simulink model "Vehicle_Speedometer_Module"  (R2022a)
settings: Solver=FixedStepDiscrete  StartTime=0.0  StopTime=10.0  FixedStep=0.01  RelTol=1e-3
libraries: simulink x1
settings Model: DataDictionary=VSM_Data_Dictionary.sldd  EnableAccessToBaseWorkspace=off  Creator=jamesbond  LastModifiedBy=jamesbond
settings OptimizationCC: DefaultParameterBehavior=Inlined  EnhancedBackFolding=on  PassReuseOutputArgsAs=Individual arguments  ZeroExternalMemoryAtStartup=off  ZeroInternalMemoryAtStartup=off  OptimizeBlockOrder=speed  DifferentSizesBufferReuse=on  OptimizationCustomize=off  EfficientTunableParamExpr=on
settings DebuggingCC: SignalInfNanChecking=error  SignalRangeChecking=warning  CheckMatrixSingularityMsg=error  IntegerOverflowMsg=none  ParameterOverflowMsg=none  ParameterTunabilityLossMsg=error  ModelReferenceVersionMismatchMessage=warning  ModelReferenceIOMismatchMessage=warning  IntegerSaturationMsg=none
settings HardwareCC: ProdBitPerLong=64  ProdHWDeviceType=Intel->x86-64 (Mac OS X)
settings SFSimCC: MATLABDynamicMemAlloc=off
settings RTWCC: SystemTargetFile=ert.tlc  TemplateMakefile=ert_default_tmf  GenerateReport=on  LaunchReport=on  GenerateCodeMetricsReport=on
settings CodeAppCC: ForceParamTrailComments=on  IgnoreCustomStorageClasses=off  OperatorAnnotations=on  SimulinkDataObjDesc=on  SFDataObjDesc=on  InsertBlockDesc=on
settings ERTTargetCC: TargetLangStandard=C99 (ISO)  GenerateSampleERTMain=on  InlinedParameterPlacement=NonHierarchical  ERTCustomFileTemplate=example_file_process.tlc
settings ConfigComp: DVMaxProcessTime=3000  DVModelCoverageObjectives=MCDC  DVTestSuiteOptimization=Auto  DVDetectDeadLogic=on  DVDetectOutOfBounds=on  DVModelReferenceHarness=on  DVHarnessSource=Signal Editor

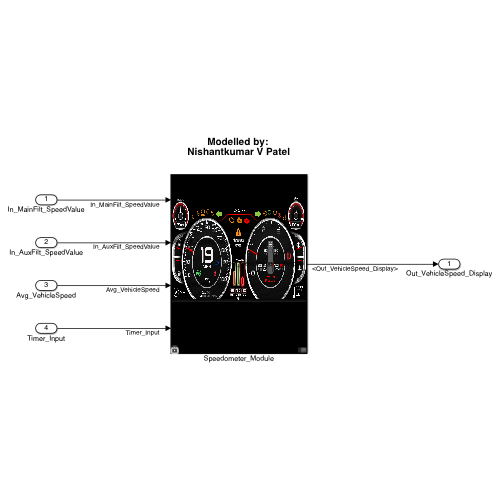
[thumbnail: Simulink's stored preview of the top-level diagram]
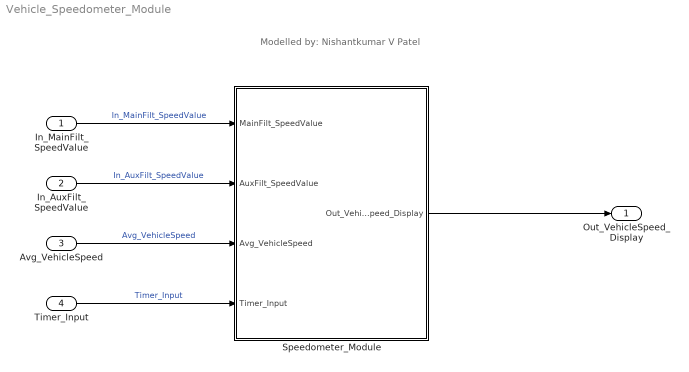
== system Vehicle_Speedometer_Module ==
  note: Modelled by:
      | Nishantkumar V Patel
  In_MainFilt_SpeedValue : Inport  OutMin=1  OutMax=3  OutDataTypeStr=fixdt(0,8,1,0)  PortDimensions=1  SampleTime=0.01
  In_AuxFilt_SpeedValue : Inport  Port=2  OutMin=1  OutMax=3  OutDataTypeStr=fixdt(0,8,1,0)  PortDimensions=1  SampleTime=0.01
  Avg_VehicleSpeed : Inport  Port=3  OutMin=0  OutMax=280  OutDataTypeStr=fixdt(0,16,0.01,0)  PortDimensions=1  SampleTime=0.01
  Timer_Input : Inport  Port=4  OutDataTypeStr=fixdt(0,16,0)  PortDimensions=1  SampleTime=0.01
  Speedometer_Module : Subsystem  TreatAsAtomicUnit=on
      mask Display: image('$imagefile'); % Use "Edit Image" on toolstrip to change.
  Out_VehicleSpeed_Display : Outport
  wires:
  Speedometer_Module/1(Out_VehicleSpeed_Display) -> Out_VehicleSpeed_Display/1
  In_MainFilt_SpeedValue/1 -> Speedometer_Module/1(MainFilt_SpeedValue)  "In_MainFilt_SpeedValue"
  In_AuxFilt_SpeedValue/1 -> Speedometer_Module/2(AuxFilt_SpeedValue)  "In_AuxFilt_SpeedValue"
  Avg_VehicleSpeed/1 -> Speedometer_Module/3(Avg_VehicleSpeed)  "Avg_VehicleSpeed"
  Timer_Input/1 -> Speedometer_Module/4(Timer_Input)  "Timer_Input"

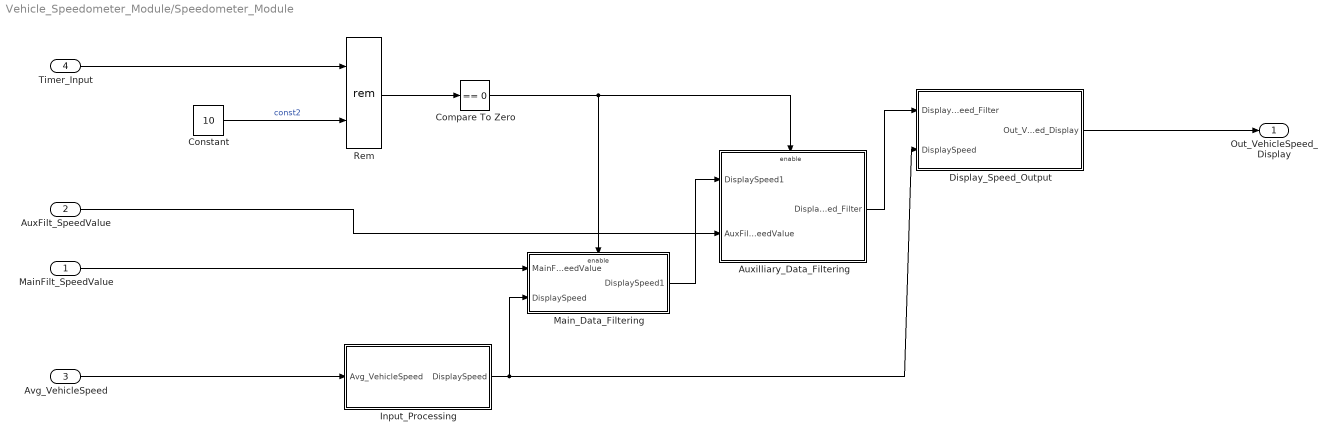
== system Vehicle_Speedometer_Module/Speedometer_Module ==
  MainFilt_SpeedValue : Inport  OutMin=1  OutMax=3  OutDataTypeStr=fixdt(0,8,1,0)  PortDimensions=1  SampleTime=0.01
  AuxFilt_SpeedValue : Inport  Port=2  OutMin=1  OutMax=3  OutDataTypeStr=fixdt(0,8,1,0)  PortDimensions=1  SampleTime=0.01
  Avg_VehicleSpeed : Inport  Port=3  OutMin=0  OutMax=280  OutDataTypeStr=fixdt(0,16,0.01,0)  PortDimensions=1  SampleTime=0.01
  Timer_Input : Inport  Port=4  OutDataTypeStr=fixdt(0,16,0)  PortDimensions=1  SampleTime=0.01
  Auxilliary_Data_Filtering : Subsystem
  Compare To Zero : simulink/Logic and Bit Operations/Compare To Zero  relop===  OutDataTypeStr=boolean
  Constant : Constant  Value=10  OutDataTypeStr=fixdt(0,16,0)
  Display_Speed_Output : Subsystem
  Input_Processing : Subsystem
  Main_Data_Filtering : Subsystem
  Rem : Math  Operator=rem
  Out_VehicleSpeed_Display : Outport
  wires:
  Avg_VehicleSpeed/1 -> Input_Processing/1(Avg_VehicleSpeed)
  MainFilt_SpeedValue/1 -> Main_Data_Filtering/1(MainFilt_SpeedValue)
  Input_Processing/1(DisplaySpeed) -> Main_Data_Filtering/2(DisplaySpeed), Display_Speed_Output/2(DisplaySpeed)
  Auxilliary_Data_Filtering/1(DisplaySpeed_Filter) -> Display_Speed_Output/1(DisplaySpeed_Filter)
  Display_Speed_Output/1(Out_VehicleSpeed_Display) -> Out_VehicleSpeed_Display/1
  Timer_Input/1 -> Rem/1
  Constant/1 -> Rem/2  "const2"
  Rem/1 -> Compare To Zero/1
  Compare To Zero/1 -> Main_Data_Filtering/Enable, Auxilliary_Data_Filtering/Enable
  Main_Data_Filtering/1(DisplaySpeed1) -> Auxilliary_Data_Filtering/1(DisplaySpeed1)
  AuxFilt_SpeedValue/1 -> Auxilliary_Data_Filtering/2(AuxFilt_SpeedValue)

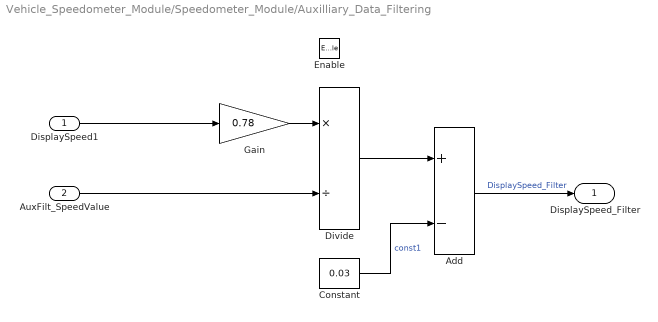
== system Vehicle_Speedometer_Module/Speedometer_Module/Auxilliary_Data_Filtering ==
  DisplaySpeed1 : Inport  OutDataTypeStr=fixdt(0,16,0.01,0)  PortDimensions=1  SampleTime=0.01
  AuxFilt_SpeedValue : Inport  Port=2
  Enable : EnablePort
  Add : Sum  Inputs=+-  AccumDataTypeStr=fixdt(0,16,0.01,0)  OutDataTypeStr=fixdt(0,16,0.01,0)
  Constant : Constant  Value=0.03  OutMin=0.03  OutMax=0.03  OutDataTypeStr=fixdt(0,16,0.01,0)
  Divide : Product  Inputs=*/  OutDataTypeStr=fixdt(0,16,0.01,0)
  Gain : Gain  Gain=0.78  ParamMin=0.78  ParamMax=0.78  ParamDataTypeStr=fixdt(0,16,0.01,0)  OutDataTypeStr=fixdt(0,16,0.01,0)
  DisplaySpeed_Filter : Outport  OutDataTypeStr=fixdt(0,16,0.01,0)  PortDimensions=1  SampleTime=0.01
  wires:
  Gain/1 -> Divide/1
  Add/1 -> DisplaySpeed_Filter/1  "DisplaySpeed_Filter"
  Constant/1 -> Add/2  "const1"
  DisplaySpeed1/1 -> Gain/1
  AuxFilt_SpeedValue/1 -> Divide/2
  Divide/1 -> Add/1

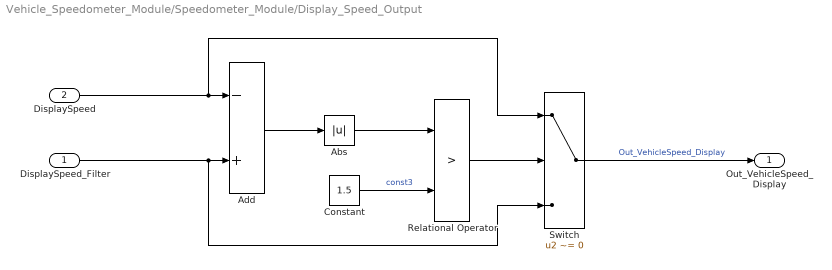
== system Vehicle_Speedometer_Module/Speedometer_Module/Display_Speed_Output ==
  DisplaySpeed_Filter : Inport  OutDataTypeStr=fixdt(0,16,0.01,0)  PortDimensions=1  SampleTime=0.01
  DisplaySpeed : Inport  Port=2  OutDataTypeStr=fixdt(0,16,0.01,0)  PortDimensions=1  SampleTime=0.01
  Abs : Abs  OutDataTypeStr=fixdt(0,16,0.01,0)  SaturateOnIntegerOverflow=off
  Add : Sum  Inputs=-+  AccumDataTypeStr=fixdt(1,16,0.01,0)  OutDataTypeStr=fixdt(1,16,0.01,0)  SaturateOnIntegerOverflow=on
  Constant : Constant  Value=1.5  OutMin=1.5  OutMax=1.5  OutDataTypeStr=fixdt(0,16,0.01,0)
  Relational Operator : RelationalOperator  Operator=>  OutDataTypeStr=boolean  RndMeth=Simplest  InputSameDT=off
  Switch : Switch  Criteria=u2 ~= 0  OutDataTypeStr=fixdt(0,16,0.01,0)  SaturateOnIntegerOverflow=off  InputSameDT=off
  Out_VehicleSpeed_Display : Outport
  wires:
  DisplaySpeed/1 -> Switch/1, Add/1
  DisplaySpeed_Filter/1 -> Add/2, Switch/3
  Add/1 -> Abs/1
  Abs/1 -> Relational Operator/1
  Constant/1 -> Relational Operator/2  "const3"
  Relational Operator/1 -> Switch/2
  Switch/1 -> Out_VehicleSpeed_Display/1  "Out_VehicleSpeed_Display"

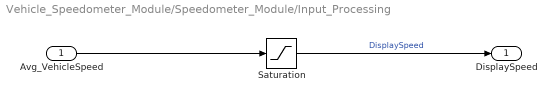
== system Vehicle_Speedometer_Module/Speedometer_Module/Input_Processing ==
  Avg_VehicleSpeed : Inport  OutMin=0  OutMax=280  OutDataTypeStr=fixdt(0,16,0.01,0)  PortDimensions=1  SampleTime=0.01
  Saturation : Saturate  UpperLimit=250  LowerLimit=2  OutDataTypeStr=fixdt(0,16,0.01,0)
  DisplaySpeed : Outport  OutDataTypeStr=fixdt(0,16,0.01,0)  PortDimensions=1  SampleTime=0.01
  wires:
  Saturation/1 -> DisplaySpeed/1  "DisplaySpeed"
  Avg_VehicleSpeed/1 -> Saturation/1

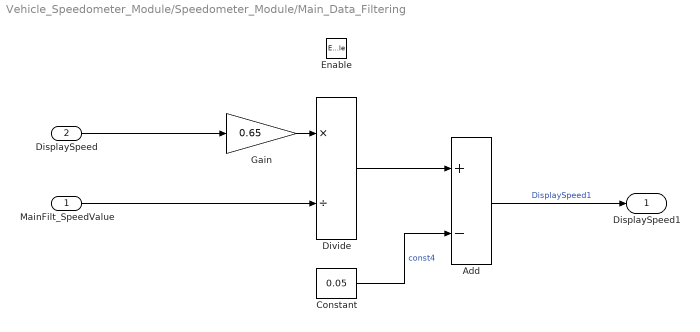
== system Vehicle_Speedometer_Module/Speedometer_Module/Main_Data_Filtering ==
  MainFilt_SpeedValue : Inport  OutMin=1  OutMax=3  OutDataTypeStr=fixdt(0,8,1,0)  PortDimensions=1  SampleTime=0.01
  DisplaySpeed : Inport  Port=2  OutDataTypeStr=fixdt(0,16,0.01,0)  PortDimensions=1  SampleTime=0.01
  Enable : EnablePort
  Add : Sum  Inputs=+-  AccumDataTypeStr=fixdt(0,16,0.01,0)  OutDataTypeStr=fixdt(0,16,0.01,0)
  Constant : Constant  Value=0.05  OutMin=0.05  OutMax=0.05  OutDataTypeStr=fixdt(0,16,0.01,0)
  Divide : Product  Inputs=*/  OutDataTypeStr=fixdt(0,16,0.01,0)
  Gain : Gain  Gain=0.65  ParamMin=0.65  ParamMax=0.65  ParamDataTypeStr=fixdt(0,16,0.01,0)  OutDataTypeStr=fixdt(0,16,0.01,0)
  DisplaySpeed1 : Outport  OutDataTypeStr=fixdt(0,16,0.01,0)  PortDimensions=1  SampleTime=0.01
  wires:
  Gain/1 -> Divide/1
  Divide/1 -> Add/1
  Add/1 -> DisplaySpeed1/1  "DisplaySpeed1"
  Constant/1 -> Add/2  "const4"
  DisplaySpeed/1 -> Gain/1
  MainFilt_SpeedValue/1 -> Divide/2
